simulink model "UTPC"  (R2022b)
settings: Solver=FixedStepAuto  StartTime=0.0  StopTime=10.0  FixedStep=1  RelTol=1e-3
undefined symbols (not defined in the file): DiscIntNeverNeededParam
libraries: simulink x3
settings Model: Creator=sadamu  LastModifiedBy=sadamu
settings OptimizationCC: DefaultParameterBehavior=Inlined  DefaultUnderspecifiedDataType=single  BufferReuse=off  GlobalBufferReuse=off  ExpressionFolding=off  EnableMemcpy=off  PassReuseOutputArgsAs=Individual arguments  NoFixptDivByZeroProtection=on  EfficientFloat2IntCast=on  OptimizeDataStoreBuffers=off  BusAssignmentInplaceUpdate=off  OptimizationLevel=level0  EfficientTunableParamExpr=on
settings DebuggingCC: ParameterTunabilityLossMsg=error
settings SFSimCC: MATLABDynamicMemAlloc=off
settings RTWCC: Description=Embedded Coder  SystemTargetFile=ert.tlc  GenCodeOnly=on  TemplateMakefile=ert_default_tmf
settings CodeAppCC: ForceParamTrailComments=on  IgnoreCustomStorageClasses=off  OperatorAnnotations=on  SimulinkDataObjDesc=on  SFDataObjDesc=on  InsertBlockDesc=on
settings ERTTargetCC: TargetLangStandard=C99 (ISO)  GenerateSampleERTMain=on  CodeInterfacePackaging=Reusable function  InlinedParameterPlacement=NonHierarchical  ERTCustomFileTemplate=example_file_process.tlc
settings ConfigComp: CovMetricSettings=dcmwe  DVMaxProcessTime=3600  DVTestSuiteOptimization=Auto  DVDetectOutOfBounds=on  DVModelReferenceHarness=on

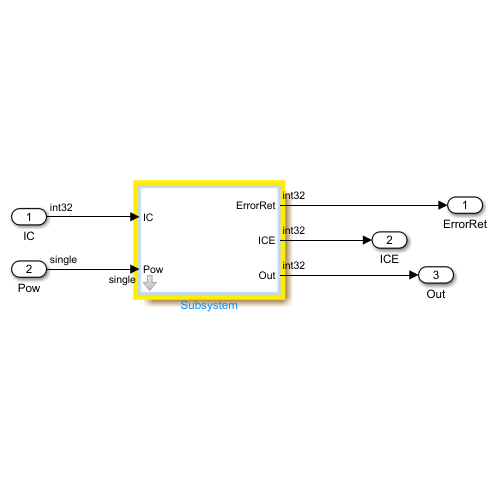
[thumbnail: Simulink's stored preview of the top-level diagram]
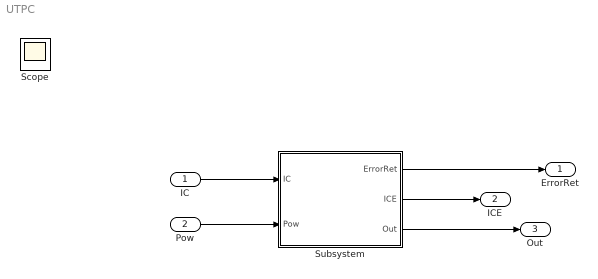
== system UTPC ==
  IC : Inport  OutDataTypeStr=int32
  Pow : Inport  Port=2  OutDataTypeStr=single
  Subsystem : Subsystem  mask{Len=40}
      mask DialogControl ParameterGroupVar Prompt: 参数
  ErrorRet : Outport
  ICE : Outport  Port=2
  Out : Outport  Port=3
  Scope : Scope
  wires:
  IC/1 -> Subsystem/1(IC)
  Pow/1 -> Subsystem/2(Pow)
  Subsystem/1(ErrorRet) -> ErrorRet/1
  Subsystem/2(ICE) -> ICE/1
  Subsystem/3(Out) -> Out/1

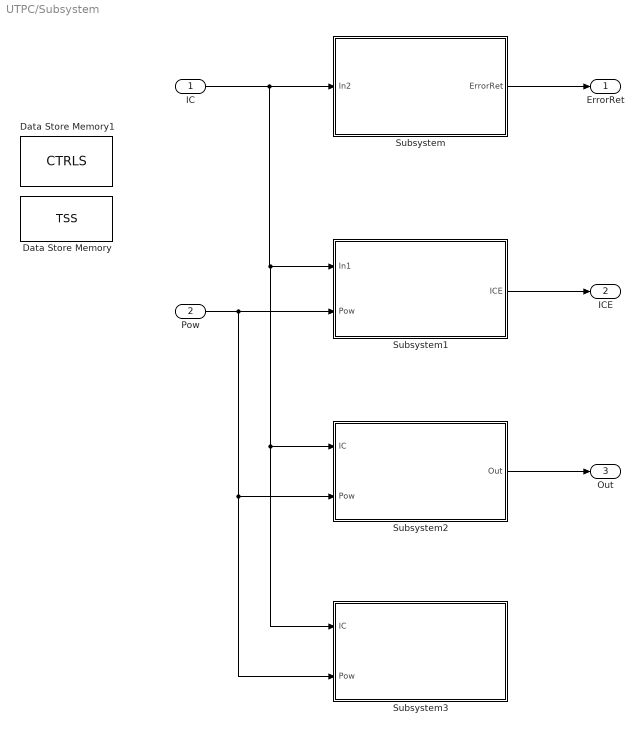
== system UTPC/Subsystem ==
  IC : Inport
  Pow : Inport  Port=2  OutDataTypeStr=single
  Data Store Memory : DataStoreMemory  DataStoreName=TSS  WriteAfterWriteMsg=warning  ShowAdditionalParam=off  OutDataTypeStr=single  Dimensions=Len
  Data Store Memory1 : DataStoreMemory  DataStoreName=CTRLS  WriteAfterWriteMsg=warning  ShowAdditionalParam=off  OutDataTypeStr=int32
  Subsystem : Subsystem
  Subsystem1 : Subsystem
  Subsystem2 : Subsystem
  Subsystem3 : Subsystem
  ErrorRet : Outport
  ICE : Outport  Port=2
  Out : Outport  Port=3
  wires:
  IC/1 -> Subsystem3/1(IC), Subsystem2/1(IC), Subsystem1/1(In1), Subsystem/1(In2)
  Subsystem/1(ErrorRet) -> ErrorRet/1
  Pow/1 -> Subsystem1/2(Pow), Subsystem3/2(Pow), Subsystem2/2(Pow)
  Subsystem1/1(ICE) -> ICE/1
  Subsystem2/1(Out) -> Out/1

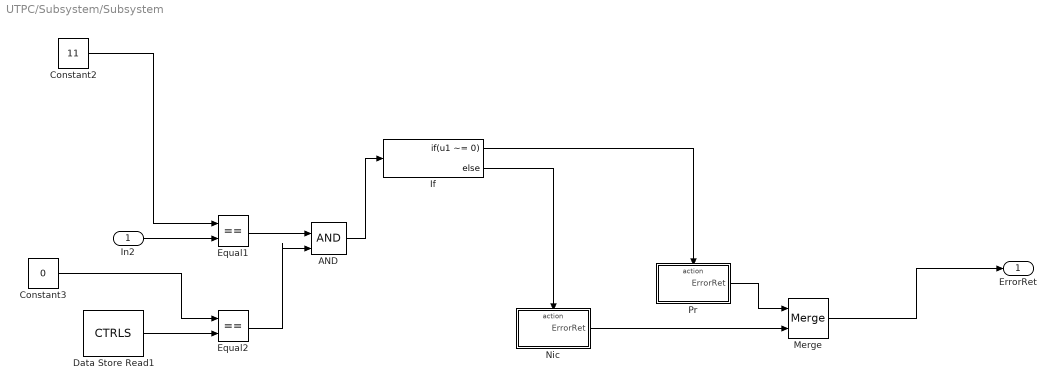
== system UTPC/Subsystem/Subsystem ==
  In2 : Inport
  AND : Logic  IconShape=distinctive  AllPortsSameDT=off  OutDataTypeStr=boolean
  Constant2 : Constant  Value=11  OutDataTypeStr=int32
  Constant3 : Constant  Value=0  OutDataTypeStr=int32
  Data Store Read1 : DataStoreRead  DataStoreName=CTRLS  IndexOptions=Index vector (dialog)  Indices=1  OutputSizes=1
  Equal1 : RelationalOperator  Operator===  OutDataTypeStr=boolean  RndMeth=Simplest  InputSameDT=off
  Equal2 : RelationalOperator  Operator===  OutDataTypeStr=boolean  RndMeth=Simplest  InputSameDT=off
  If : If  IfExpression=u1 ~= 0
  Merge : Merge
  Nic : Subsystem  TreatAsAtomicUnit=on
  Pr : Subsystem  TreatAsAtomicUnit=on
  ErrorRet : Outport
  wires:
  Data Store Read1/1 -> Equal2/2
  Constant2/1 -> Equal1/1
  Pr/1(ErrorRet) -> Merge/1
  Equal1/1 -> AND/1
  Equal2/1 -> AND/2
  If/1 -> Pr/Action
  AND/1 -> If/1
  If/2 -> Nic/Action
  Constant3/1 -> Equal2/1
  Nic/1(ErrorRet) -> Merge/2
  In2/1 -> Equal1/2
  Merge/1 -> ErrorRet/1

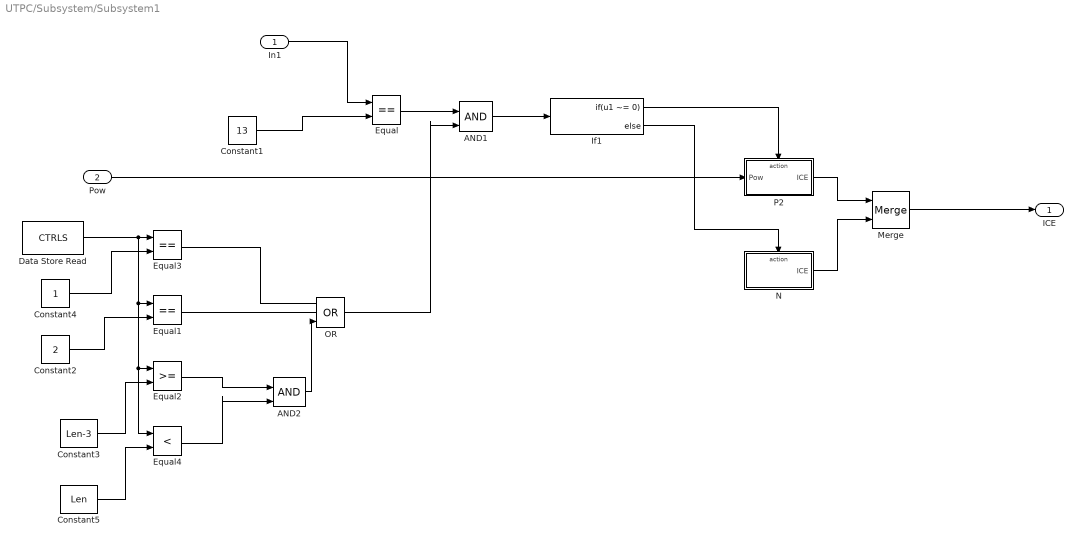
== system UTPC/Subsystem/Subsystem1 ==
  In1 : Inport
  Pow : Inport  Port=2
  AND1 : Logic  IconShape=distinctive  AllPortsSameDT=off  OutDataTypeStr=boolean
  AND2 : Logic  IconShape=distinctive  AllPortsSameDT=off  OutDataTypeStr=boolean
  Constant1 : Constant  Value=13  OutDataTypeStr=int32
  Constant2 : Constant  Value=2  OutDataTypeStr=int32
  Constant3 : Constant  Value=Len-3  OutDataTypeStr=int32
  Constant4 : Constant  OutDataTypeStr=int32
  Constant5 : Constant  Value=Len  OutDataTypeStr=int32
  Data Store Read : DataStoreRead  DataStoreName=CTRLS  IndexOptions=Index vector (dialog)  Indices=1  OutputSizes=1
  Equal : RelationalOperator  Operator===  OutDataTypeStr=boolean  RndMeth=Simplest  InputSameDT=off
  Equal1 : RelationalOperator  Operator===  OutDataTypeStr=boolean  RndMeth=Simplest  InputSameDT=off
  Equal2 : RelationalOperator  OutDataTypeStr=boolean  RndMeth=Simplest  InputSameDT=off
  Equal3 : RelationalOperator  Operator===  OutDataTypeStr=boolean  RndMeth=Simplest  InputSameDT=off
  Equal4 : RelationalOperator  Operator=<  OutDataTypeStr=boolean  RndMeth=Simplest  InputSameDT=off
  If1 : If  IfExpression=u1 ~= 0
  Merge : Merge
  N : Subsystem  TreatAsAtomicUnit=on
  OR : Logic  Operator=OR  Inputs=3  IconShape=distinctive  AllPortsSameDT=off  OutDataTypeStr=boolean
  P2 : Subsystem  TreatAsAtomicUnit=on
  ICE : Outport
  wires:
  Data Store Read/1 -> Equal1/1, Equal4/1, Equal2/1, Equal3/1
  AND1/1 -> If1/1
  N/1(ICE) -> Merge/2
  Equal3/1 -> OR/1
  Constant1/1 -> Equal/2
  Equal/1 -> AND1/1
  If1/1 -> P2/Action
  If1/2 -> N/Action
  P2/1(ICE) -> Merge/1
  Constant4/1 -> Equal3/2
  Pow/1 -> P2/1(Pow)
  In1/1 -> Equal/1
  Merge/1 -> ICE/1
  Constant2/1 -> Equal1/2
  Constant3/1 -> Equal2/2
  Constant5/1 -> Equal4/2
  Equal4/1 -> AND2/2
  Equal2/1 -> AND2/1
  AND2/1 -> OR/3
  Equal1/1 -> OR/2
  OR/1 -> AND1/2

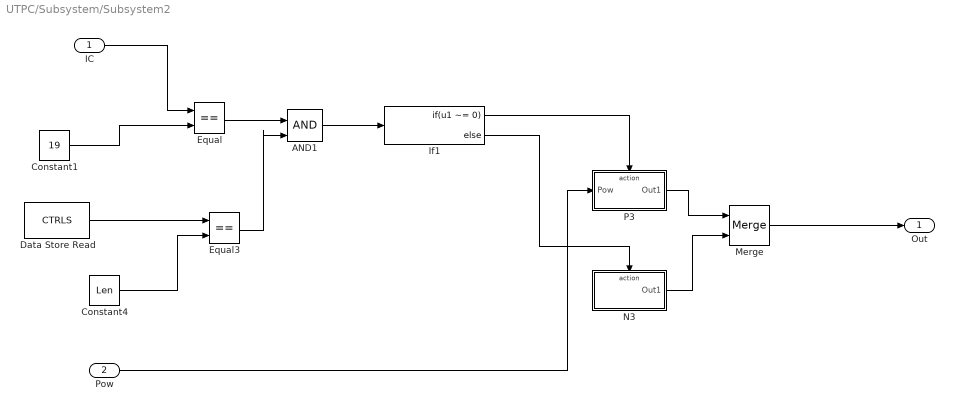
== system UTPC/Subsystem/Subsystem2 ==
  IC : Inport
  Pow : Inport  Port=2
  AND1 : Logic  IconShape=distinctive  AllPortsSameDT=off  OutDataTypeStr=boolean
  Constant1 : Constant  Value=19  OutDataTypeStr=int32
  Constant4 : Constant  Value=Len  OutDataTypeStr=int32
  Data Store Read : DataStoreRead  DataStoreName=CTRLS  IndexOptions=Index vector (dialog)  Indices=1  OutputSizes=1
  Equal : RelationalOperator  Operator===  OutDataTypeStr=boolean  RndMeth=Simplest  InputSameDT=off
  Equal3 : RelationalOperator  Operator===  OutDataTypeStr=boolean  RndMeth=Simplest  InputSameDT=off
  If1 : If  IfExpression=u1 ~= 0
  Merge : Merge
  N3 : Subsystem  TreatAsAtomicUnit=on
  P3 : Subsystem  TreatAsAtomicUnit=on
  Out : Outport
  wires:
  Data Store Read/1 -> Equal3/1
  AND1/1 -> If1/1
  N3/1(Out1) -> Merge/2
  Equal3/1 -> AND1/2
  Constant1/1 -> Equal/2
  Equal/1 -> AND1/1
  If1/1 -> P3/Action
  If1/2 -> N3/Action
  P3/1(Out1) -> Merge/1
  Constant4/1 -> Equal3/2
  IC/1 -> Equal/1
  Merge/1 -> Out/1
  Pow/1 -> P3/1(Pow)

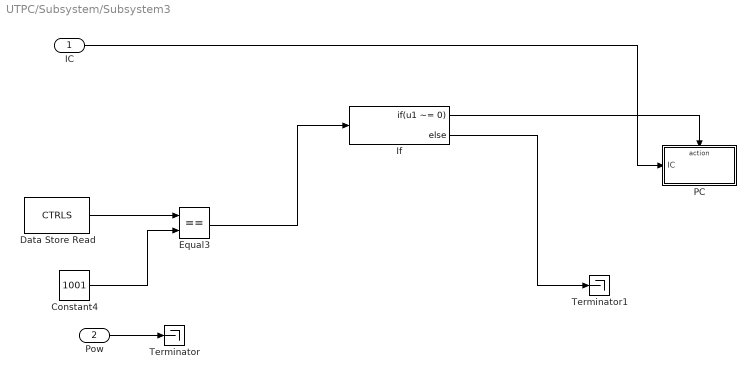
== system UTPC/Subsystem/Subsystem3 ==
  IC : Inport
  Pow : Inport  Port=2
  Constant4 : Constant  Value=1001  OutDataTypeStr=int32
  Data Store Read : DataStoreRead  DataStoreName=CTRLS  IndexOptions=Index vector (dialog)  Indices=1  OutputSizes=1
  Equal3 : RelationalOperator  Operator===  OutDataTypeStr=boolean  RndMeth=Simplest  InputSameDT=off
  If : If  IfExpression=u1 ~= 0
  PC : Subsystem  TreatAsAtomicUnit=on
  Terminator : Terminator
  Terminator1 : Terminator
  wires:
  Data Store Read/1 -> Equal3/1
  Constant4/1 -> Equal3/2
  Pow/1 -> Terminator/1
  If/2 -> Terminator1/1
  If/1 -> PC/Action
  Equal3/1 -> If/1
  IC/1 -> PC/1(IC)

== system UTPC/Subsystem/Subsystem/Nic ==
  Action Port : ActionPort  ActionPortLabel=else
  Constant : Constant  Value=-1  OutDataTypeStr=int32
  ErrorRet : Outport
  wires:
  Constant/1 -> ErrorRet/1

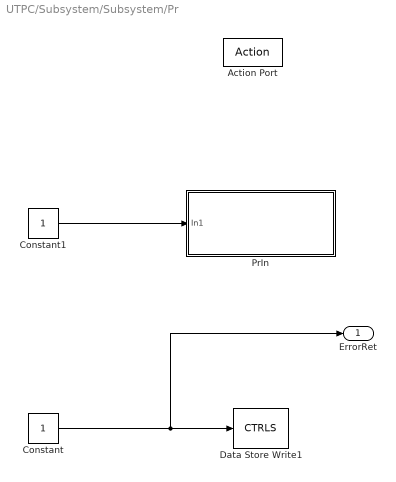
== system UTPC/Subsystem/Subsystem/Pr ==
  Action Port : ActionPort  ActionPortLabel=if(u1 ~= 0)
  Constant : Constant  OutDataTypeStr=int32
  Constant1 : Constant  OutDataTypeStr=single
  Data Store Write1 : DataStoreWrite  DataStoreName=CTRLS  IndexOptions=Index vector (dialog)  Indices=1  OutputSizes=1
  PrIn : Subsystem  TreatAsAtomicUnit=on
  ErrorRet : Outport
  wires:
  Constant/1 -> ErrorRet/1, Data Store Write1/1
  Constant1/1 -> PrIn/1(In1)

== system UTPC/Subsystem/Subsystem1/N ==
  Action Port : ActionPort  ActionPortLabel=else
  Constant4 : Constant  Value=2  OutDataTypeStr=int32
  ICE : Outport
  wires:
  Constant4/1 -> ICE/1

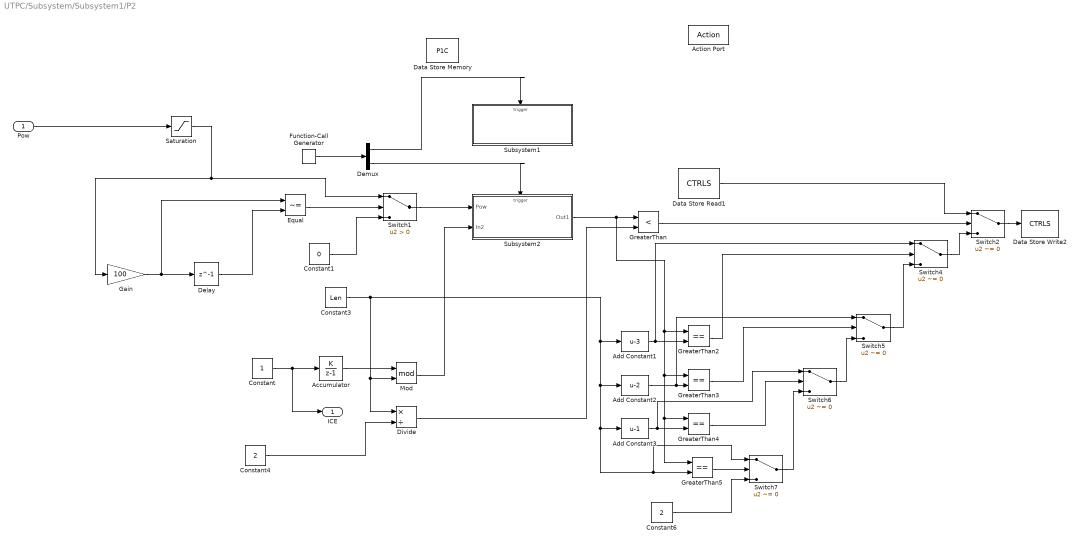
== system UTPC/Subsystem/Subsystem1/P2 ==
  Pow : Inport
  Action Port : ActionPort  ActionPortLabel=if(u1 ~= 0)
  Accumulator : DiscreteIntegrator  IntegratorMethod=Accumulation: Forward Euler  SampleTime=-1  ICPrevOutput=DiscIntNeverNeededParam  ICPrevScaledInput=DiscIntNeverNeededParam
  Add Constant1 : Bias  Bias=-3  SaturateOnIntegerOverflow=off
  Add Constant2 : Bias  Bias=-2  SaturateOnIntegerOverflow=off
  Add Constant3 : Bias  Bias=-1  SaturateOnIntegerOverflow=off
  Constant : Constant  OutDataTypeStr=int32
  Constant1 : Constant  Value=0  OutDataTypeStr=single
  Constant3 : Constant  Value=Len  OutDataTypeStr=int32
  Constant4 : Constant  Value=2  OutDataTypeStr=int32
  Constant6 : Constant  Value=2  OutDataTypeStr=int32
  Data Store Memory : DataStoreMemory  DataStoreName=P1C  WriteAfterWriteMsg=warning  ShowAdditionalParam=off  OutDataTypeStr=int32
  Data Store Read1 : DataStoreRead  DataStoreName=CTRLS  IndexOptions=Index vector (dialog)  Indices=1  OutputSizes=1
  Data Store Write2 : DataStoreWrite  DataStoreName=CTRLS  IndexOptions=Index vector (dialog)  Indices=1  OutputSizes=1
  Delay : Delay  DelayLength=1
  Demux : Demux  Outputs=2
  Divide : Product  Inputs=*/
  Equal : RelationalOperator  Operator=~=  OutDataTypeStr=boolean  RndMeth=Simplest  InputSameDT=off
  Function-Call Generator : simulink/Ports & Subsystems/Function-Call Generator  sample_time=1  numberOfIterations=1  DisallowWideOutput=off
  Gain : Gain  Gain=100  OutDataTypeStr=int32
  GreaterThan : RelationalOperator  Operator=<  OutDataTypeStr=boolean  RndMeth=Simplest  InputSameDT=off
  GreaterThan{2..5} (4 alike) : RelationalOperator  Operator===  OutDataTypeStr=boolean  RndMeth=Simplest  InputSameDT=off
  Mod : Math  Operator=mod
  Saturation : Saturate  UpperLimit=4  LowerLimit=1
  Subsystem1 : Subsystem
  Subsystem2 : Subsystem
  Switch1 : Switch  Criteria=u2 > Threshold  SaturateOnIntegerOverflow=off  InputSameDT=off
  Switch{2,4..7} (5 alike) : Switch  Criteria=u2 ~= 0  SaturateOnIntegerOverflow=off  InputSameDT=off
  ICE : Outport
  wires:
  Constant/1 -> ICE/1, Accumulator/1
  Mod/1 -> Subsystem2/2(In2)
  Pow/1 -> Saturation/1
  Saturation/1 -> Gain/1, Switch1/1
  Gain/1 -> Equal/1, Delay/1
  Equal/1 -> Switch1/2
  Constant1/1 -> Switch1/3
  Demux/2 -> Subsystem2/Trigger
  Demux/1 -> Subsystem1/Trigger
  Function-Call Generator/1 -> Demux/1
  Constant3/1 -> Switch7/1, GreaterThan5/2, Add Constant3/1, Add Constant2/1, Add Constant1/1, Mod/2, Divide/1
  Divide/1 -> GreaterThan/2
  Constant4/1 -> Divide/2
  Accumulator/1 -> Mod/1
  Delay/1 -> Equal/2
  Switch1/1 -> Subsystem2/1(Pow)
  Data Store Read1/1 -> Switch2/1
  Switch2/1 -> Data Store Write2/1
  GreaterThan/1 -> Switch2/2
  Add Constant1/1 -> Switch4/1, GreaterThan2/2
  GreaterThan2/1 -> Switch4/2
  Switch4/1 -> Switch2/3
  Add Constant2/1 -> Switch5/1, GreaterThan3/2
  GreaterThan3/1 -> Switch5/2
  GreaterThan4/1 -> Switch6/2
  Subsystem2/1(Out1) -> GreaterThan5/1, GreaterThan4/1, GreaterThan3/1, GreaterThan2/1, GreaterThan/1
  Add Constant3/1 -> Switch6/1, GreaterThan4/2
  GreaterThan5/1 -> Switch7/2
  Constant6/1 -> Switch7/3
  Switch5/1 -> Switch4/3
  Switch6/1 -> Switch5/3
  Switch7/1 -> Switch6/3

== system UTPC/Subsystem/Subsystem2/N3 ==
  Action Port : ActionPort  ActionPortLabel=else
  Constant4 : Constant  Value=-2  OutDataTypeStr=int32
  Out1 : Outport
  wires:
  Constant4/1 -> Out1/1

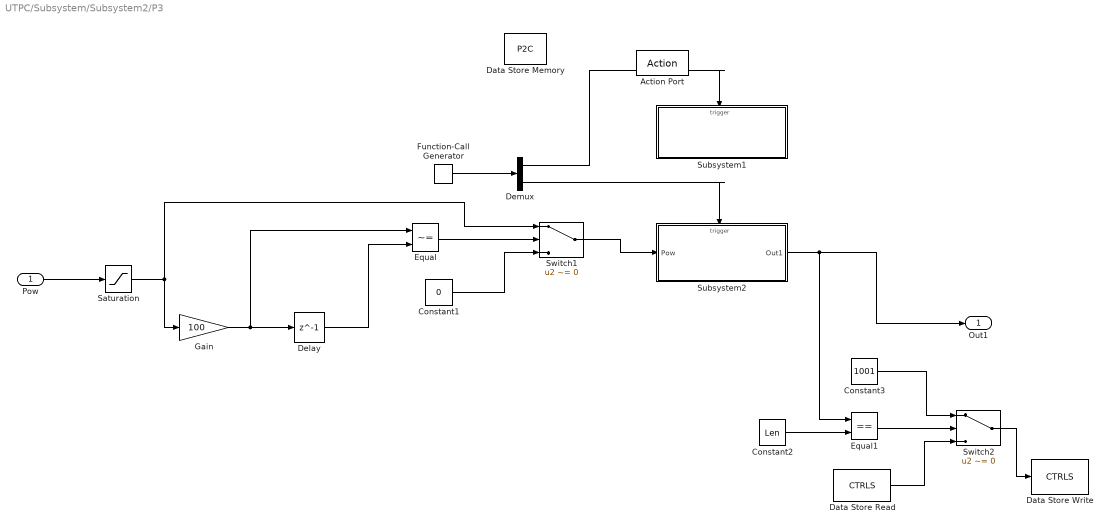
== system UTPC/Subsystem/Subsystem2/P3 ==
  Pow : Inport
  Action Port : ActionPort  ActionPortLabel=if(u1 ~= 0)
  Constant1 : Constant  Value=0  OutDataTypeStr=single
  Constant2 : Constant  Value=Len  OutDataTypeStr=int32
  Constant3 : Constant  Value=1001  OutDataTypeStr=int32
  Data Store Memory : DataStoreMemory  DataStoreName=P2C  WriteAfterWriteMsg=warning  ShowAdditionalParam=off  OutDataTypeStr=int32
  Data Store Read : DataStoreRead  DataStoreName=CTRLS  IndexOptions=Index vector (dialog)  Indices=1  OutputSizes=1
  Data Store Write : DataStoreWrite  DataStoreName=CTRLS  IndexOptions=Index vector (dialog)  Indices=1  OutputSizes=1
  Delay : Delay  DelayLength=1
  Demux : Demux  Outputs=2
  Equal : RelationalOperator  Operator=~=  OutDataTypeStr=boolean  RndMeth=Simplest  InputSameDT=off
  Equal1 : RelationalOperator  Operator===  OutDataTypeStr=boolean  RndMeth=Simplest  InputSameDT=off
  Function-Call Generator : simulink/Ports & Subsystems/Function-Call Generator  sample_time=1  numberOfIterations=1  DisallowWideOutput=off
  Gain : Gain  Gain=100  OutDataTypeStr=int32
  Saturation : Saturate  UpperLimit=1.2  LowerLimit=0.5
  Subsystem1 : Subsystem
  Subsystem2 : Subsystem
  Switch1 : Switch  Criteria=u2 ~= 0  SaturateOnIntegerOverflow=off  InputSameDT=off
  Switch2 : Switch  Criteria=u2 ~= 0  SaturateOnIntegerOverflow=off  InputSameDT=off
  Out1 : Outport
  wires:
  Pow/1 -> Saturation/1
  Saturation/1 -> Gain/1, Switch1/1
  Gain/1 -> Equal/1, Delay/1
  Equal/1 -> Switch1/2
  Constant1/1 -> Switch1/3
  Delay/1 -> Equal/2
  Switch1/1 -> Subsystem2/1(Pow)
  Subsystem2/1(Out1) -> Equal1/1, Out1/1
  Function-Call Generator/1 -> Demux/1
  Demux/1 -> Subsystem1/Trigger
  Demux/2 -> Subsystem2/Trigger
  Constant2/1 -> Equal1/2
  Equal1/1 -> Switch2/2
  Constant3/1 -> Switch2/1
  Data Store Read/1 -> Switch2/3
  Switch2/1 -> Data Store Write/1

== system UTPC/Subsystem/Subsystem3/PC ==
  IC : Inport
  Action Port : ActionPort  ActionPortLabel=if(u1 ~= 0)
  Constant1 : Constant  Value=10.0  OutDataTypeStr=single
  PrIn : Subsystem  TreatAsAtomicUnit=on
  wires:
  Constant1/1 -> PrIn/1(In1)
  IC/1 -> PrIn/2(IC)

== system UTPC/Subsystem/Subsystem/Pr/PrIn ==
  In1 : Inport
  Assignment : Assignment  IndexMode=Zero-based  DiagnosticForDimensions=Warning  IndexOptions=Index vector (port)  Indices=1  OutputSizes=1
  Data Store Read : DataStoreRead  DataStoreName=TSS  IndexOptions=Index vector (dialog)  Indices=1  OutputSizes=1
  Data Store Write : DataStoreWrite  DataStoreName=TSS  IndexOptions=Index vector (dialog)  Indices=1  OutputSizes=1
  For Iterator : ForIterator  IterationLimit=Len  IndexMode=Zero-based
  wires:
  In1/1 -> Assignment/2
  For Iterator/1 -> Assignment/3
  Assignment/1 -> Data Store Write/1
  Data Store Read/1 -> Assignment/1

== system UTPC/Subsystem/Subsystem1/P2/Subsystem1 ==
  Trigger : TriggerPort  TriggerType=function-call  VariantControl=(inherit)  PortDimensions=1
  Constant : Constant  Value=0  OutDataTypeStr=int32
  Data Store Write : DataStoreWrite  DataStoreName=P1C  IndexOptions=Index vector (dialog)  Indices=1  OutputSizes=1
  wires:
  Constant/1 -> Data Store Write/1

== system UTPC/Subsystem/Subsystem1/P2/Subsystem2 ==
  Pow : Inport
  In2 : Inport  Port=2
  Trigger : TriggerPort  TriggerType=function-call  VariantControl=(inherit)  PortDimensions=1
  PF : Subsystem  TreatAsAtomicUnit=on
  Out1 : Outport
  wires:
  In2/1 -> PF/2(In1)
  Pow/1 -> PF/1(Pow)
  PF/1(Out1) -> Out1/1

== system UTPC/Subsystem/Subsystem2/P3/Subsystem1 ==
  Trigger : TriggerPort  TriggerType=function-call  VariantControl=(inherit)  PortDimensions=1
  Constant : Constant  Value=0  OutDataTypeStr=int32
  Data Store Write : DataStoreWrite  DataStoreName=P2C  IndexOptions=Index vector (dialog)  Indices=1  OutputSizes=1
  wires:
  Constant/1 -> Data Store Write/1

== system UTPC/Subsystem/Subsystem2/P3/Subsystem2 ==
  Pow : Inport
  Trigger : TriggerPort  TriggerType=function-call  VariantControl=(inherit)  PortDimensions=1
  PF : Subsystem  TreatAsAtomicUnit=on
  Out1 : Outport
  wires:
  Pow/1 -> PF/1(Pow)
  PF/1(Out1) -> Out1/1

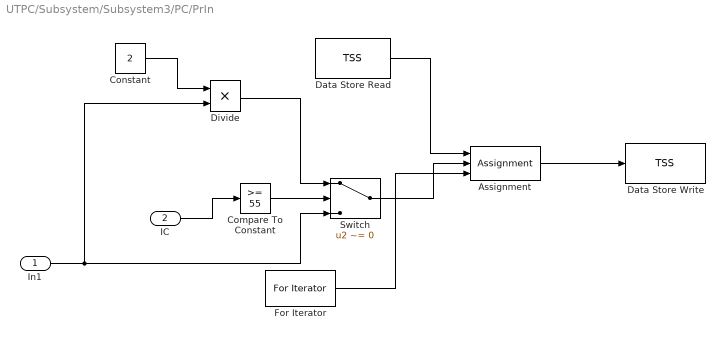
== system UTPC/Subsystem/Subsystem3/PC/PrIn ==
  In1 : Inport
  IC : Inport  Port=2
  Assignment : Assignment  IndexMode=Zero-based  DiagnosticForDimensions=Warning  IndexOptions=Index vector (port)  Indices=1  OutputSizes=1
  Compare To Constant : simulink/Logic and Bit Operations/Compare To Constant  relop=>=  const=55  OutDataTypeStr=boolean
  Constant : Constant  Value=2  OutDataTypeStr=single
  Data Store Read : DataStoreRead  DataStoreName=TSS  IndexOptions=Index vector (dialog)  Indices=1  OutputSizes=1
  Data Store Write : DataStoreWrite  DataStoreName=TSS  IndexOptions=Index vector (dialog)  Indices=1  OutputSizes=1
  Divide : Product  Inputs=**
  For Iterator : ForIterator  IterationLimit=Len  IndexMode=Zero-based
  Switch : Switch  Criteria=u2 ~= 0  SaturateOnIntegerOverflow=off  InputSameDT=off
  wires:
  In1/1 -> Divide/2, Switch/3
  For Iterator/1 -> Assignment/3
  Assignment/1 -> Data Store Write/1
  Data Store Read/1 -> Assignment/1
  IC/1 -> Compare To Constant/1
  Compare To Constant/1 -> Switch/2
  Constant/1 -> Divide/1
  Divide/1 -> Switch/1
  Switch/1 -> Assignment/2

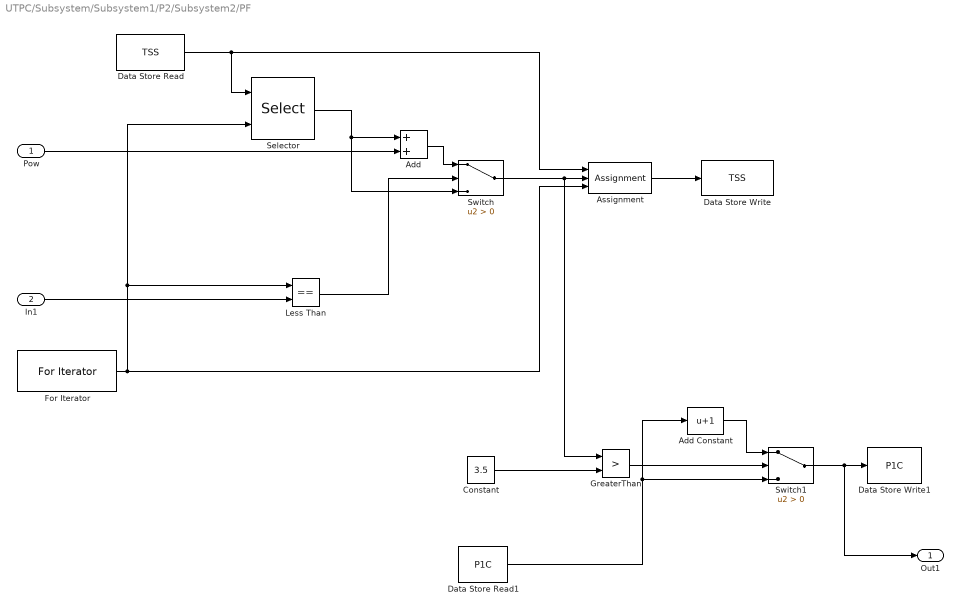
== system UTPC/Subsystem/Subsystem1/P2/Subsystem2/PF ==
  Pow : Inport
  In1 : Inport  Port=2
  Add : Sum
  Add Constant : Bias  Bias=1  SaturateOnIntegerOverflow=off
  Assignment : Assignment  IndexMode=Zero-based  DiagnosticForDimensions=Warning  IndexOptions=Index vector (port)  Indices=1  OutputSizes=1
  Constant : Constant  Value=3.5  OutDataTypeStr=single
  Data Store Read : DataStoreRead  DataStoreName=TSS  IndexOptions=Index vector (dialog)  Indices=1  OutputSizes=1
  Data Store Read1 : DataStoreRead  DataStoreName=P1C  IndexOptions=Index vector (dialog)  Indices=1  OutputSizes=1
  Data Store Write : DataStoreWrite  DataStoreName=TSS  IndexOptions=Index vector (dialog)  Indices=1  OutputSizes=1
  Data Store Write1 : DataStoreWrite  DataStoreName=P1C  IndexOptions=Index vector (dialog)  Indices=1  OutputSizes=1
  For Iterator : ForIterator  IterationLimit=Len  IndexMode=Zero-based
  GreaterThan : RelationalOperator  Operator=>  OutDataTypeStr=boolean  RndMeth=Simplest  InputSameDT=off
  Less Than : RelationalOperator  Operator===  OutDataTypeStr=boolean  RndMeth=Simplest  InputSameDT=off
  Selector : Selector  IndexMode=Zero-based  InputPortWidth=Len  IndexOptions=Index vector (port)  Indices=[1 3]  OutputSizes=1
  Switch : Switch  Criteria=u2 > Threshold  SaturateOnIntegerOverflow=off  InputSameDT=off
  Switch1 : Switch  Criteria=u2 > Threshold  SaturateOnIntegerOverflow=off  InputSameDT=off
  Out1 : Outport
  wires:
  For Iterator/1 -> Assignment/3, Less Than/1, Selector/2
  Data Store Read/1 -> Selector/1, Assignment/1
  Selector/1 -> Add/1, Switch/3
  Switch/1 -> GreaterThan/1, Assignment/2
  Pow/1 -> Add/2
  In1/1 -> Less Than/2
  Less Than/1 -> Switch/2
  Assignment/1 -> Data Store Write/1
  Add/1 -> Switch/1
  Constant/1 -> GreaterThan/2
  GreaterThan/1 -> Switch1/2
  Data Store Read1/1 -> Add Constant/1, Switch1/3
  Add Constant/1 -> Switch1/1
  Switch1/1 -> Out1/1, Data Store Write1/1

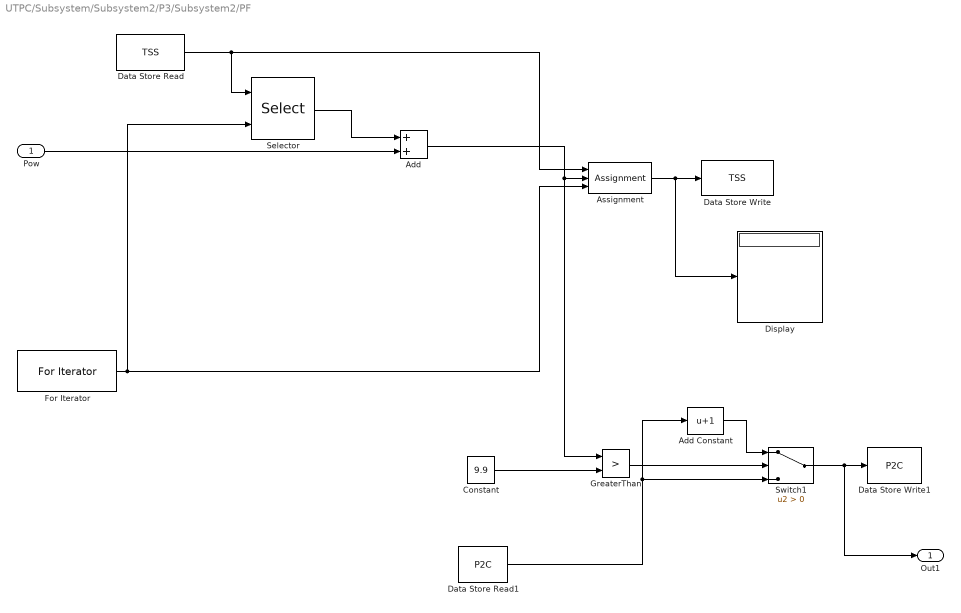
== system UTPC/Subsystem/Subsystem2/P3/Subsystem2/PF ==
  Pow : Inport
  Add : Sum
  Add Constant : Bias  Bias=1  SaturateOnIntegerOverflow=off
  Assignment : Assignment  IndexMode=Zero-based  DiagnosticForDimensions=Warning  IndexOptions=Index vector (port)  Indices=1  OutputSizes=1
  Constant : Constant  Value=9.9  OutDataTypeStr=single
  Data Store Read : DataStoreRead  DataStoreName=TSS  IndexOptions=Index vector (dialog)  Indices=1  OutputSizes=1
  Data Store Read1 : DataStoreRead  DataStoreName=P2C  IndexOptions=Index vector (dialog)  Indices=1  OutputSizes=1
  Data Store Write : DataStoreWrite  DataStoreName=TSS  IndexOptions=Index vector (dialog)  Indices=1  OutputSizes=1
  Data Store Write1 : DataStoreWrite  DataStoreName=P2C  IndexOptions=Index vector (dialog)  Indices=1  OutputSizes=1
  Display : Display
  For Iterator : ForIterator  IterationLimit=Len  IndexMode=Zero-based
  GreaterThan : RelationalOperator  Operator=>  OutDataTypeStr=boolean  RndMeth=Simplest  InputSameDT=off
  Selector : Selector  IndexMode=Zero-based  InputPortWidth=Len  IndexOptions=Index vector (port)  Indices=[1 3]  OutputSizes=1
  Switch1 : Switch  Criteria=u2 > Threshold  SaturateOnIntegerOverflow=off  InputSameDT=off
  Out1 : Outport
  wires:
  For Iterator/1 -> Assignment/3, Selector/2
  Data Store Read/1 -> Selector/1, Assignment/1
  Selector/1 -> Add/1
  Add/1 -> GreaterThan/1, Assignment/2
  Pow/1 -> Add/2
  Assignment/1 -> Display/1, Data Store Write/1
  Constant/1 -> GreaterThan/2
  GreaterThan/1 -> Switch1/2
  Data Store Read1/1 -> Add Constant/1, Switch1/3
  Add Constant/1 -> Switch1/1
  Switch1/1 -> Out1/1, Data Store Write1/1
